simulink model "Testing_Model"  (R2021b)
settings: Solver=FixedStepAuto  StartTime=0.0  StopTime=200  FixedStep=0.001  RelTol=1e-3
settings Model: Creator=Alireza  LastModifiedBy=Alireza

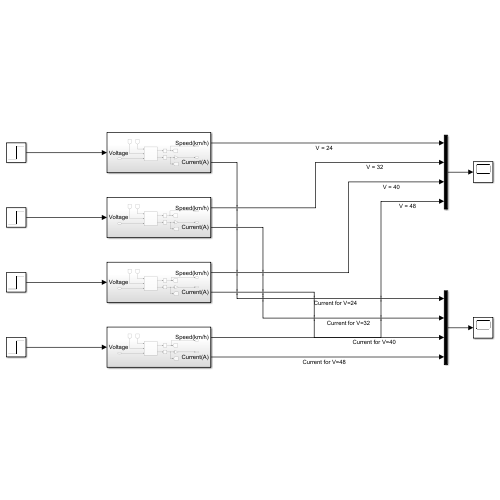
[thumbnail: Simulink's stored preview of the top-level diagram]
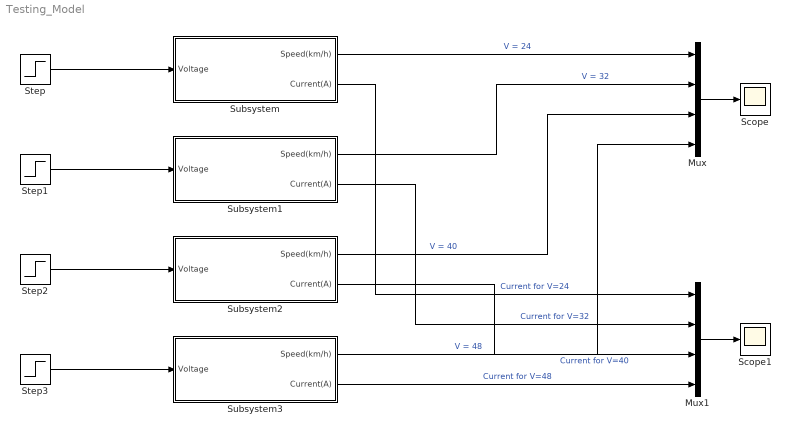
== system Testing_Model ==
  Mux : Mux
  Mux1 : Mux
  Scope : Scope
  Scope1 : Scope
  Step : Step  Time=0  After=24  SampleTime=0
  Step1 : Step  Time=0  After=32  SampleTime=0
  Step2 : Step  Time=0  After=40  SampleTime=0
  Step3 : Step  Time=0  After=48  SampleTime=0
  Subsystem : Subsystem
  Subsystem1 : Subsystem
  Subsystem2 : Subsystem
  Subsystem3 : Subsystem
  wires:
  Step3/1 -> Subsystem3/1("Voltage ")
  Step/1 -> Subsystem/1("Voltage ")
  Step1/1 -> Subsystem1/1("Voltage ")
  Step2/1 -> Subsystem2/1("Voltage ")
  Subsystem/1(Speed(km/h)) -> Mux/1  "V = 24"
  Subsystem1/1(Speed(km/h)) -> Mux/2  "V = 32"
  Subsystem2/1(Speed(km/h)) -> Mux/3  "V = 40"
  Subsystem3/1(Speed(km/h)) -> Mux/4  "V = 48"
  Mux/1 -> Scope/1
  Subsystem3/2(Current(A)) -> Mux1/4  "Current for V=48"
  Subsystem2/2(Current(A)) -> Mux1/3  "Current for V=40"
  Subsystem1/2(Current(A)) -> Mux1/2  "Current for V=32"
  Subsystem/2(Current(A)) -> Mux1/1  "Current for V=24"
  Mux1/1 -> Scope1/1

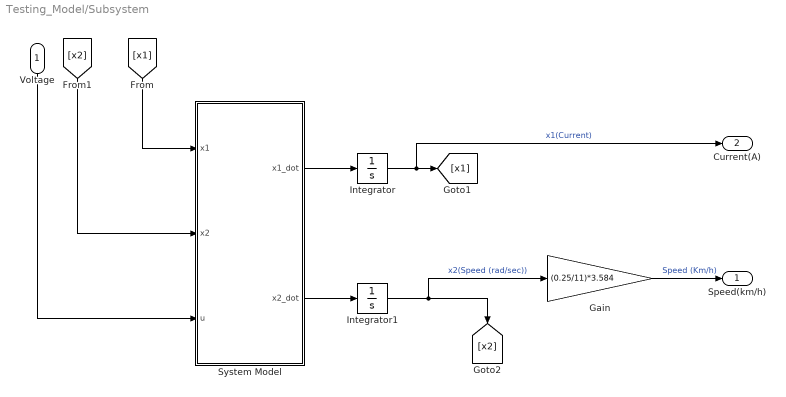
== system Testing_Model/Subsystem ==
  "Voltage " : Inport
  Gain : Gain  Gain=(0.25/11)*3.584
  Integrator : Integrator  InitialCondition=5
  Integrator1 : Integrator
  System Model : MATLAB Function  TreatAsAtomicUnit=on
  Speed(km/h) : Outport
  Current(A) : Outport  Port=2
  wires:
  System Model/1(x1_dot) -> Integrator/1
  Integrator1/1 -> Gain/1, [x2]  "x2(Speed (rad/sec))"
  System Model/2(x2_dot) -> Integrator1/1
  [x2] -> System Model/2(x2)
  [x1] -> System Model/1(x1)
  Gain/1 -> Speed(km/h)/1  "Speed (Km/h)"
  Integrator/1 -> Current(A)/1, [x1]  "x1(Current)"
  "Voltage "/1 -> System Model/3(u)

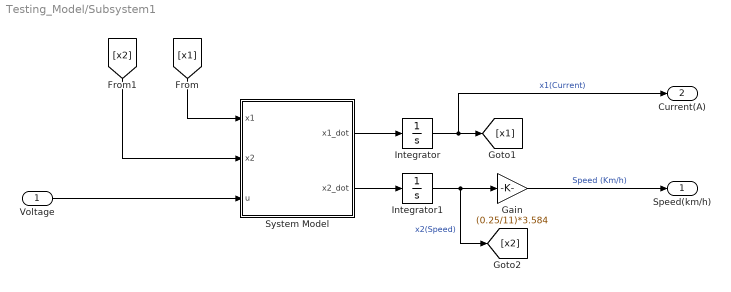
== system Testing_Model/Subsystem1 ==
  "Voltage " : Inport
  Gain : Gain  Gain=(0.25/11)*3.584
  Integrator : Integrator  InitialCondition=5
  Integrator1 : Integrator
  System Model : MATLAB Function  TreatAsAtomicUnit=on
  Speed(km/h) : Outport
  Current(A) : Outport  Port=2
  wires:
  System Model/1(x1_dot) -> Integrator/1
  Integrator1/1 -> [x2], Gain/1  "x2(Speed)"
  System Model/2(x2_dot) -> Integrator1/1
  [x2] -> System Model/2(x2)
  [x1] -> System Model/1(x1)
  Gain/1 -> Speed(km/h)/1  "Speed (Km/h)"
  Integrator/1 -> Current(A)/1, [x1]  "x1(Current)"
  "Voltage "/1 -> System Model/3(u)

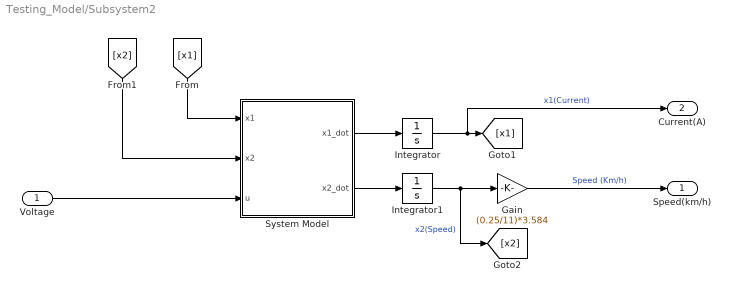
== system Testing_Model/Subsystem2 ==
  "Voltage " : Inport
  Gain : Gain  Gain=(0.25/11)*3.584
  Integrator : Integrator  InitialCondition=5
  Integrator1 : Integrator
  System Model : MATLAB Function  TreatAsAtomicUnit=on
  Speed(km/h) : Outport
  Current(A) : Outport  Port=2
  wires:
  System Model/1(x1_dot) -> Integrator/1
  Integrator1/1 -> [x2], Gain/1  "x2(Speed)"
  System Model/2(x2_dot) -> Integrator1/1
  [x2] -> System Model/2(x2)
  [x1] -> System Model/1(x1)
  Gain/1 -> Speed(km/h)/1  "Speed (Km/h)"
  Integrator/1 -> Current(A)/1, [x1]  "x1(Current)"
  "Voltage "/1 -> System Model/3(u)

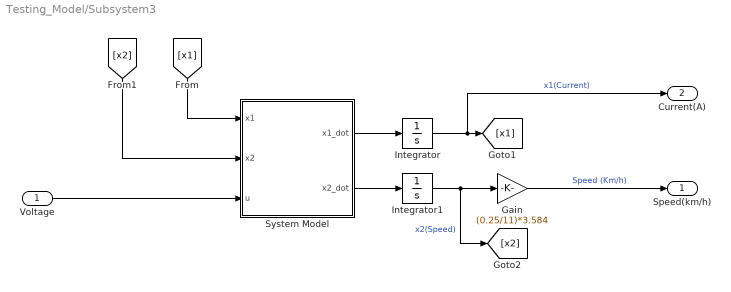
== system Testing_Model/Subsystem3 ==
  "Voltage " : Inport
  Gain : Gain  Gain=(0.25/11)*3.584
  Integrator : Integrator  InitialCondition=5
  Integrator1 : Integrator
  System Model : MATLAB Function  TreatAsAtomicUnit=on
  Speed(km/h) : Outport
  Current(A) : Outport  Port=2
  wires:
  System Model/1(x1_dot) -> Integrator/1
  Integrator1/1 -> [x2], Gain/1  "x2(Speed)"
  System Model/2(x2_dot) -> Integrator1/1
  [x2] -> System Model/2(x2)
  [x1] -> System Model/1(x1)
  Gain/1 -> Speed(km/h)/1  "Speed (Km/h)"
  Integrator/1 -> Current(A)/1, [x1]  "x1(Current)"
  "Voltage "/1 -> System Model/3(u)

== matlab function Testing_Model/Subsystem1/System Model ==
  data: x1 input; x1_dot output; x2 input; u input; x2_dot output
function [x1_dot, x2_dot]= fcn(x1, x2, u)
Ra_plus_Rf = 0.12;      % Armature and Field Resistance
La_plus_Lf = 6.008e-3;  % Armature and Field Inductance
r = 0.25;               % Wheel Radious
J = 0.05;               % Inertai of the Motor
L_af = 1.766e-3;        % Mutual Inductance
I = 78;                 % Maximum Current
omega_norm = 2800;      % Nominal omega
m = 800;                % Total mass (kg)
A = 1.8;                % Frontal Area of the Vegicle
ro = 1.25;              % Air density
Cd = 0.3;               % Drag Coefficient
phi = 0;                % Hill climbing Angle
mu_rr = 0.015;          % Rolling Resistance Coefficient
G = 11;                 % Gearbox Ratio
B = 0.0002;             % Viscous Coefficient
g = 9.8;                % Gravity Constant 
V = 48;                 % Input Voltage  0 ~ 48 volt

x1_dot = (1/La_plus_Lf) * (-(Ra_plus_Rf) * x1 - L_af * x1 * x2) + (1/La_plus_Lf) * u;
x2_dot = (1 / (J + m * (r/G)^2)) * (L_af * x1^2 -B * x2 - (r/G) * (mu_rr * m * g + 0.5 * ro * A * Cd * (r/G)^2 * x2^2 + m*g*sin(phi)));


end

== matlab function Testing_Model/Subsystem/System Model ==
  data: x1 input; x1_dot output; x2 input; u input; x2_dot output
function [x1_dot, x2_dot]= fcn(x1, x2, u)
Ra_plus_Rf = 0.12;      % Armature and Field Resistance
La_plus_Lf = 6.008e-3;  % Armature and Field Inductance
r = 0.25;               % Wheel Radious
J = 0.05;               % Inertai of the Motor
L_af = 1.766e-3;        % Mutual Inductance
I = 78;                 % Maximum Current
omega_norm = 2800;      % Nominal omega
m = 800;                % Total mass (kg)
A = 1.8;                % Frontal Area of the Vegicle
ro = 1.25;              % Air density
Cd = 0.3;               % Drag Coefficient
phi = 0;                % Hill climbing Angle
mu_rr = 0.015;          % Rolling Resistance Coefficient
G = 11;                 % Gearbox Ratio
B = 0.0002;             % Viscous Coefficient
g = 9.8;                % Gravity Constant 
V = 48;                 % Input Voltage  0 ~ 48 volt

x1_dot = (1/La_plus_Lf) * (-(Ra_plus_Rf) * x1 - L_af * x1 * x2) + (1/La_plus_Lf) * u;
x2_dot = (1 / (J + m * (r/G)^2)) * (L_af * x1^2 -B * x2 - (r/G) * (mu_rr * m * g + 0.5 * ro * A * Cd * (r/G)^2 * x2^2 + m*g*sin(phi)));


end

== matlab function Testing_Model/Subsystem2/System Model ==
  data: x1 input; x1_dot output; x2 input; u input; x2_dot output
function [x1_dot, x2_dot]= fcn(x1, x2, u)
Ra_plus_Rf = 0.12;      % Armature and Field Resistance
La_plus_Lf = 6.008e-3;  % Armature and Field Inductance
r = 0.25;               % Wheel Radious
J = 0.05;               % Inertai of the Motor
L_af = 1.766e-3;        % Mutual Inductance
I = 78;                 % Maximum Current
omega_norm = 2800;      % Nominal omega
m = 800;                % Total mass (kg)
A = 1.8;                % Frontal Area of the Vegicle
ro = 1.25;              % Air density
Cd = 0.3;               % Drag Coefficient
phi = 0;                % Hill climbing Angle
mu_rr = 0.015;          % Rolling Resistance Coefficient
G = 11;                 % Gearbox Ratio
B = 0.0002;             % Viscous Coefficient
g = 9.8;                % Gravity Constant 
V = 48;                 % Input Voltage  0 ~ 48 volt

x1_dot = (1/La_plus_Lf) * (-(Ra_plus_Rf) * x1 - L_af * x1 * x2) + (1/La_plus_Lf) * u;
x2_dot = (1 / (J + m * (r/G)^2)) * (L_af * x1^2 -B * x2 - (r/G) * (mu_rr * m * g + 0.5 * ro * A * Cd * (r/G)^2 * x2^2 + m*g*sin(phi)));


end

== matlab function Testing_Model/Subsystem3/System Model ==
  data: x1 input; x1_dot output; x2 input; u input; x2_dot output
function [x1_dot, x2_dot]= fcn(x1, x2, u)
Ra_plus_Rf = 0.12;      % Armature and Field Resistance
La_plus_Lf = 6.008e-3;  % Armature and Field Inductance
r = 0.25;               % Wheel Radious
J = 0.05;               % Inertai of the Motor
L_af = 1.766e-3;        % Mutual Inductance
I = 78;                 % Maximum Current
omega_norm = 2800;      % Nominal omega
m = 800;                % Total mass (kg)
A = 1.8;                % Frontal Area of the Vegicle
ro = 1.25;              % Air density
Cd = 0.3;               % Drag Coefficient
phi = 0;                % Hill climbing Angle
mu_rr = 0.015;          % Rolling Resistance Coefficient
G = 11;                 % Gearbox Ratio
B = 0.0002;             % Viscous Coefficient
g = 9.8;                % Gravity Constant 
V = 48;                 % Input Voltage  0 ~ 48 volt

x1_dot = (1/La_plus_Lf) * (-(Ra_plus_Rf) * x1 - L_af * x1 * x2) + (1/La_plus_Lf) * u;
x2_dot = (1 / (J + m * (r/G)^2)) * (L_af * x1^2 -B * x2 - (r/G) * (mu_rr * m * g + 0.5 * ro * A * Cd * (r/G)^2 * x2^2 + m*g*sin(phi)));


end
